simulink model "s_sip_freefall_ss_vs_eom"  (Simulink 6.6)
settings: Solver=ode4  StartTime=0.0  StopTime=3  FixedStep=0.002  RelTol=1e-3  AbsTol=1e-6
values from neighbouring files (symbols this model uses):
  A = handles.A    [d_gui_lqr_tuning.m]
  B = handles.B    [d_gui_lqr_tuning.m]
  Beq = 5.4    [setup_ip01_2_configuration.m]
  C = handles.C    [d_gui_lqr_tuning.m]    (also in d_ip01_2_sip_lqr.m = eye( 4 ))
  D = handles.D    [d_gui_lqr_tuning.m]    (also in d_ip01_2_sip_lqr.m = zeros( 4, 1 ))
  Eff_g = 1    [setup_ip01_2_configuration.m]
  Eff_m = 1    [setup_ip01_2_configuration.m]
  IC_ALPHA0 = IC_ALPHA0 / 180 * pi    (= 0)    [setup_lab_ip01_2_sip.m]
  IMAX_AMP = 1.6    [setup_ip01_2_configuration.m]
  Kg = 3.71    [setup_ip01_2_configuration.m]
  Km = 0.804e-3 * K_RDPS2RPM    [setup_ip01_2_configuration.m]
  Kt = 1.088 * K_OZ2N * K_IN2M    [setup_ip01_2_configuration.m]
  Mc = Mc + Eff_g * Kg^2 * Jm / r_mp^2    [setup_lab_ip01_2_sip.m]
  r_mp = 0.5 / 2 * K_IN2M    [setup_ip01_2_configuration.m]
  Rm = 2.6    [setup_ip01_2_configuration.m]
undefined symbols (not defined in the file or in its folder): Bp, g, Ip, lp, Mp
libraries: simulink_extras x1
settings Model: Creator=MLevis  LastModifiedBy=MLevis  ExtModeTrigDuration=5000  ExtModeArmWhenConnect=off  BufferReuse=off
settings SolverCC: PositivePriorityOrder=on
settings DataIOCC: LimitDataPoints=off
settings OptimizationCC: BooleanDataType=off  OptimizeBlockIOStorage=off  BufferReuse=off  EnforceIntegerDowncast=off  ExpressionFolding=off  FoldNonRolledExpr=off  LocalBlockOutputs=off
settings DebuggingCC: SignalResolutionControl=TryResolveAllWithWarning  SolverPrmCheckMsg=none  MultiTaskDSMMsg=warning  MultiTaskCondExecSysMsg=none  StrictBusMsg=None
settings RTWCC: SystemTargetFile=quarc_windows.tlc  TemplateMakefile=quarc_default_tmf  Description=QUARC Win32 Target  ProcessScript=quarc_windows_make_rtw_hook  IncludeERTFirstTime=on
settings STFCustomTargetCC: TargetFcnLib=ansi_tfl_tmw.mat  TargetPreCompLibLocation=C:\DOCUME~1\ALLUSE~1\APPLIC~1\QUARC\lib\2007a\windows\release  GenFloatMathFcnCalls=ANSI_C  SystemTargetFile=quarc_windows.tlc
settings GRTTargetCC: TargetPreCompLibLocation=C:\DOCUME~1\ALLUSE~1\APPLIC~1\QUARC\lib\2007a\windows\release  MatFileLogging=off  ExtMode=on  ExtModeMexFile=quarc_comm

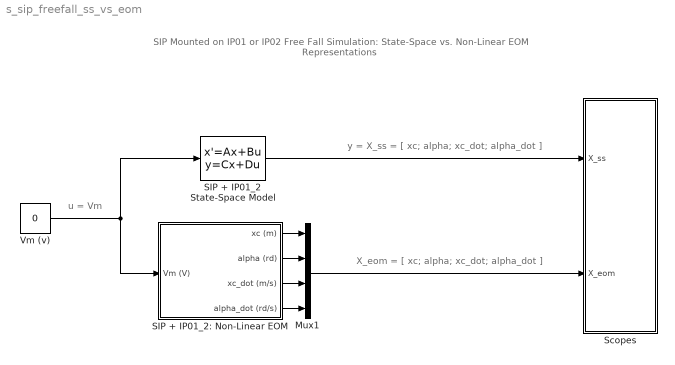
== system s_sip_freefall_ss_vs_eom ==
  note: SIP Mounted on IP01 or IP02
      | Free Fall Simulation:
      | State-Space vs. Non-Linear EOM Representations
  note: u = Vm
  note: y = X_ss = [ xc; alpha; xc_dot; alpha_dot ]
  note: X_eom = [ xc; alpha; xc_dot; alpha_dot ]
  Mux1 : Mux
  SIP + IP01_2 State-Space Model : StateSpace  A=A  B=B  C=C  D=D  X0=[ 0; IC_ALPHA0; 0; 0 ]
  SIP + IP01_2: Non-Linear EOM : Subsystem
  Scopes : Subsystem
  Vm (v) : Constant  Value=0
  wires:
  Vm (v)/1 -> SIP + IP01_2 State-Space Model/1, SIP + IP01_2: Non-Linear EOM/1(Vm (V))
  Mux1/1 -> Scopes/2(X_eom)
  SIP + IP01_2 State-Space Model/1 -> Scopes/1(X_ss)
  SIP + IP01_2: Non-Linear EOM/1(xc (m)) -> Mux1/1
  SIP + IP01_2: Non-Linear EOM/2(alpha (rd)) -> Mux1/2
  SIP + IP01_2: Non-Linear EOM/3(xc_dot (m/s)) -> Mux1/3
  SIP + IP01_2: Non-Linear EOM/4(alpha_dot (rd/s)) -> Mux1/4

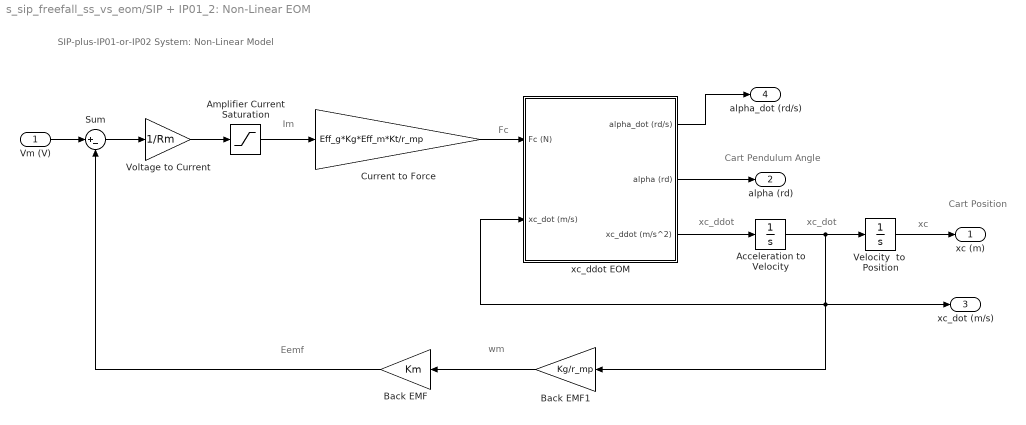
== system s_sip_freefall_ss_vs_eom/SIP + IP01_2: Non-Linear EOM ==
  note: SIP-plus-IP01-or-IP02 System:
      | Non-Linear Model
  note: Fc
  note: Im
  note: Eemf
  note: wm
  note: xc_dot
  note: xc_ddot
  note: xc
  note: Cart Position
  note: Cart Pendulum Angle
  Vm (V) : Inport
  Acceleration to Velocity : Integrator
  Amplifier Current Saturation : Saturate  UpperLimit=IMAX_AMP  LowerLimit=- IMAX_AMP
  Back EMF : Gain  Orientation=left  Gain=Km  SaturateOnIntegerOverflow=on
  Back EMF1 : Gain  Orientation=left  Gain=Kg/r_mp  SaturateOnIntegerOverflow=on
  Current to Force : Gain  Gain=Eff_g*Kg*Eff_m*Kt/r_mp  SaturateOnIntegerOverflow=on
  Sum : Sum  Inputs=|+-  SaturateOnIntegerOverflow=on  InputSameDT=on
  Velocity  to  Position : Integrator
  Voltage to Current : Gain  Gain=1/Rm  SaturateOnIntegerOverflow=on
  xc_ddot EOM : Subsystem
  xc (m) : Outport
  alpha (rd) : Outport  Port=2
  xc_dot (m/s) : Outport  Port=3  InitialOutput=0
  alpha_dot (rd/s) : Outport  Port=4  InitialOutput=0
  wires:
  Sum/1 -> Voltage to Current/1
  Voltage to Current/1 -> Amplifier Current Saturation/1
  Acceleration to Velocity/1 -> xc_dot (m/s)/1, xc_ddot EOM/2(xc_dot (m/s)), Back EMF1/1, Velocity  to  Position/1
  Back EMF1/1 -> Back EMF/1
  Vm (V)/1 -> Sum/1
  Velocity  to  Position/1 -> xc (m)/1
  Back EMF/1 -> Sum/2
  Amplifier Current Saturation/1 -> Current to Force/1
  Current to Force/1 -> xc_ddot EOM/1(Fc (N))
  xc_ddot EOM/3(xc_ddot (m/s^2)) -> Acceleration to Velocity/1
  xc_ddot EOM/1(alpha_dot (rd/s)) -> alpha_dot (rd/s)/1
  xc_ddot EOM/2(alpha (rd)) -> alpha (rd)/1

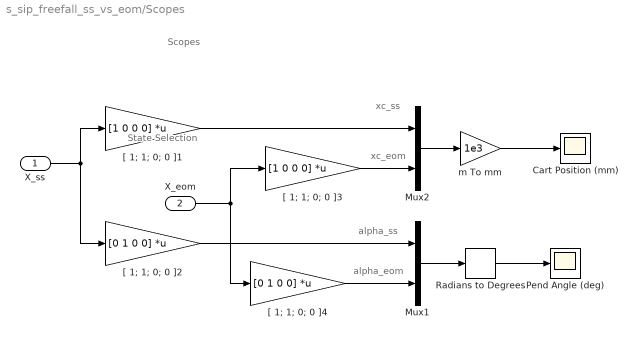
== system s_sip_freefall_ss_vs_eom/Scopes ==
  note: xc_ss
  note: State Selection
  note: alpha_ss
  note: alpha_eom
  note: xc_eom
  note: Scopes
  X_ss : Inport
  X_eom : Inport  Port=2
  Cart Position (mm) : Scope
      settings: TickLabels=on  TimeRange=3  YMin=-50  YMax=50  DataFormat=Array
  Mux1 : Mux  Inputs=2
  Mux2 : Mux  Inputs=2
  Pend Angle (deg) : Scope
      settings: TickLabels=on  TimeRange=3  YMin=-2  YMax=320  DataFormat=Array
  Radians to Degrees : simulink_extras/Transformations/Radians to Degrees  SystemSampleTime=-1
  "[ 1; 1; 0; 0 ]1" : Gain  Gain=[1 0 0 0]  Multiplication=Matrix(K*u)  SaturateOnIntegerOverflow=on
  "[ 1; 1; 0; 0 ]2" : Gain  Gain=[0 1 0 0]  Multiplication=Matrix(K*u)  SaturateOnIntegerOverflow=on
  "[ 1; 1; 0; 0 ]3" : Gain  Gain=[1 0 0 0]  Multiplication=Matrix(K*u)  SaturateOnIntegerOverflow=on
  "[ 1; 1; 0; 0 ]4" : Gain  Gain=[0 1 0 0]  Multiplication=Matrix(K*u)  SaturateOnIntegerOverflow=on
  m To mm : Gain  Gain=1e3  SaturateOnIntegerOverflow=on
  wires:
  Mux2/1 -> m To mm/1
  m To mm/1 -> Cart Position (mm)/1
  X_ss/1 -> "[ 1; 1; 0; 0 ]1"/1, "[ 1; 1; 0; 0 ]2"/1
  Mux1/1 -> Radians to Degrees/1
  Radians to Degrees/1 -> Pend Angle (deg)/1
  X_eom/1 -> "[ 1; 1; 0; 0 ]3"/1, "[ 1; 1; 0; 0 ]4"/1
  "[ 1; 1; 0; 0 ]3"/1 -> Mux2/2
  "[ 1; 1; 0; 0 ]4"/1 -> Mux1/2
  "[ 1; 1; 0; 0 ]2"/1 -> Mux1/1
  "[ 1; 1; 0; 0 ]1"/1 -> Mux2/1

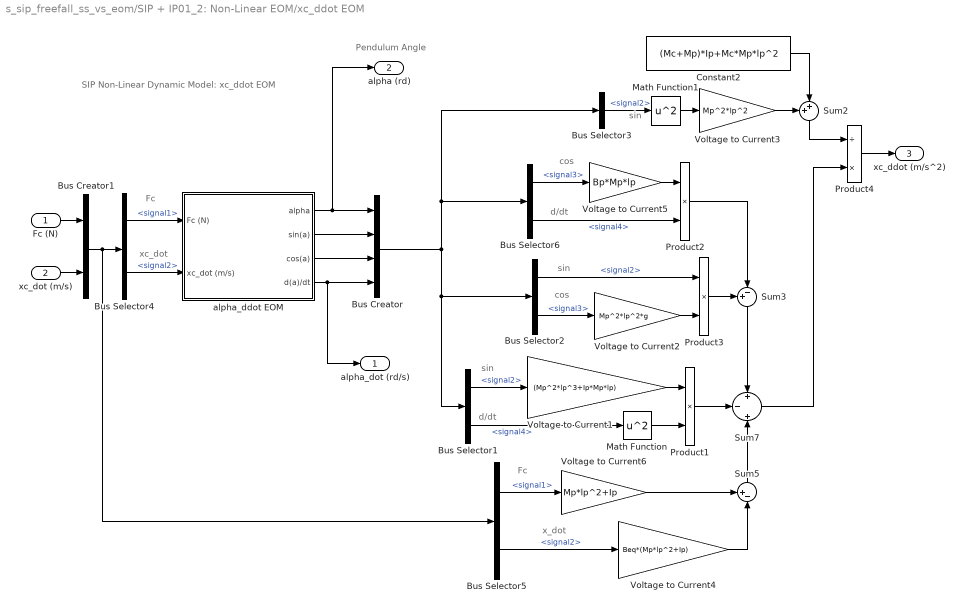
== system s_sip_freefall_ss_vs_eom/SIP + IP01_2: Non-Linear EOM/xc_ddot EOM ==
  note: xc_dot
  note: Fc
  note: x_dot
  note: Fc
  note: d/dt
  note: cos
  note: Pendulum Angle
  note: sin
  note: cos
  note: sin
  note: sin
  note: d/dt
  note: SIP Non-Linear Dynamic Model:
      | xc_ddot EOM
  Fc (N) : Inport
  xc_dot (m/s) : Inport  Port=2
  Bus Creator : BusCreator
  Bus Creator1 : BusCreator  Inputs=2
  Bus Selector1 : BusSelector  OutputSignals=signal2,signal4
  Bus Selector2 : BusSelector  OutputSignals=signal2,signal3
  Bus Selector3 : BusSelector  OutputSignals=signal2
  Bus Selector4 : BusSelector  OutputSignals=signal1,signal2
  Bus Selector5 : BusSelector  OutputSignals=signal1,signal2
  Bus Selector6 : BusSelector  OutputSignals=signal3,signal4
  Constant2 : Constant  Value=(Mc+Mp)*Ip+Mc*Mp*lp^2
  Math Function : Math  Operator=square  SaturateOnIntegerOverflow=on
  Math Function1 : Math  Operator=square  SaturateOnIntegerOverflow=on
  Product1 : Product  SaturateOnIntegerOverflow=on  RndMeth=Zero  InputSameDT=on
  Product2 : Product  SaturateOnIntegerOverflow=on  RndMeth=Zero  InputSameDT=on
  Product3 : Product  SaturateOnIntegerOverflow=on  RndMeth=Zero  InputSameDT=on
  Product4 : Product  Inputs=/*  SaturateOnIntegerOverflow=on  RndMeth=Zero  InputSameDT=on
  Sum2 : Sum  Orientation=down  Inputs=++|  SaturateOnIntegerOverflow=on  InputSameDT=on
  Sum3 : Sum  Orientation=down  Inputs=+-|  SaturateOnIntegerOverflow=on  InputSameDT=on
  Sum5 : Sum  Orientation=up  Inputs=+-|  SaturateOnIntegerOverflow=on  InputSameDT=on
  Sum7 : Sum  Inputs=+|-|+  SaturateOnIntegerOverflow=on  InputSameDT=on
  Voltage to Current1 : Gain  Gain=(Mp^2*lp^3+Ip*Mp*lp)  SaturateOnIntegerOverflow=on
  Voltage to Current2 : Gain  Gain=Mp^2*lp^2*g  SaturateOnIntegerOverflow=on
  Voltage to Current3 : Gain  Gain=Mp^2*lp^2  SaturateOnIntegerOverflow=on
  Voltage to Current4 : Gain  Gain=Beq*(Mp*lp^2+Ip)  SaturateOnIntegerOverflow=on
  Voltage to Current5 : Gain  Gain=Bp*Mp*lp  SaturateOnIntegerOverflow=on
  Voltage to Current6 : Gain  Gain=Mp*lp^2+Ip  SaturateOnIntegerOverflow=on
  alpha_ddot EOM : Subsystem
  alpha_dot (rd/s) : Outport
  alpha (rd) : Outport  Port=2
  xc_ddot (m/s^2) : Outport  Port=3
  wires:
  Voltage to Current4/1 -> Sum5/2
  Voltage to Current6/1 -> Sum5/1
  Sum5/1 -> Sum7/3
  Sum3/1 -> Sum7/1
  Product3/1 -> Sum3/1
  Product2/1 -> Sum3/2
  Sum7/1 -> Product4/2
  Bus Selector5/2 -> Voltage to Current4/1  "<signal2>"
  Bus Selector5/1 -> Voltage to Current6/1  "<signal1>"
  Voltage to Current5/1 -> Product2/1
  Bus Selector2/2 -> Voltage to Current2/1  "<signal3>"
  Bus Selector2/1 -> Product3/1  "<signal2>"
  Bus Selector6/2 -> Product2/2  "<signal4>"
  Bus Selector6/1 -> Voltage to Current5/1  "<signal3>"
  Bus Selector1/1 -> Voltage to Current1/1  "<signal2>"
  Bus Selector1/2 -> Math Function/1  "<signal4>"
  Bus Selector4/2 -> alpha_ddot EOM/2(xc_dot (m/s))  "<signal2>"
  Bus Selector4/1 -> alpha_ddot EOM/1(Fc (N))  "<signal1>"
  Bus Creator1/1 -> Bus Selector5/1, Bus Selector4/1
  xc_dot (m/s)/1 -> Bus Creator1/2
  Fc (N)/1 -> Bus Creator1/1
  alpha_ddot EOM/4(d(a)/dt) -> Bus Creator/4, alpha_dot (rd/s)/1
  alpha_ddot EOM/3(cos(a)) -> Bus Creator/3
  alpha_ddot EOM/2(sin(a)) -> Bus Creator/2
  alpha_ddot EOM/1(alpha) -> alpha (rd)/1, Bus Creator/1
  Product4/1 -> xc_ddot (m/s^2)/1
  Product1/1 -> Sum7/2
  Constant2/1 -> Sum2/2
  Voltage to Current3/1 -> Sum2/1
  Math Function1/1 -> Voltage to Current3/1
  Bus Selector3/1 -> Math Function1/1  "<signal2>"
  Voltage to Current2/1 -> Product3/2
  Math Function/1 -> Product1/2
  Voltage to Current1/1 -> Product1/1
  Bus Creator/1 -> Bus Selector6/1, Bus Selector3/1, Bus Selector1/1, Bus Selector2/1
  Sum2/1 -> Product4/1

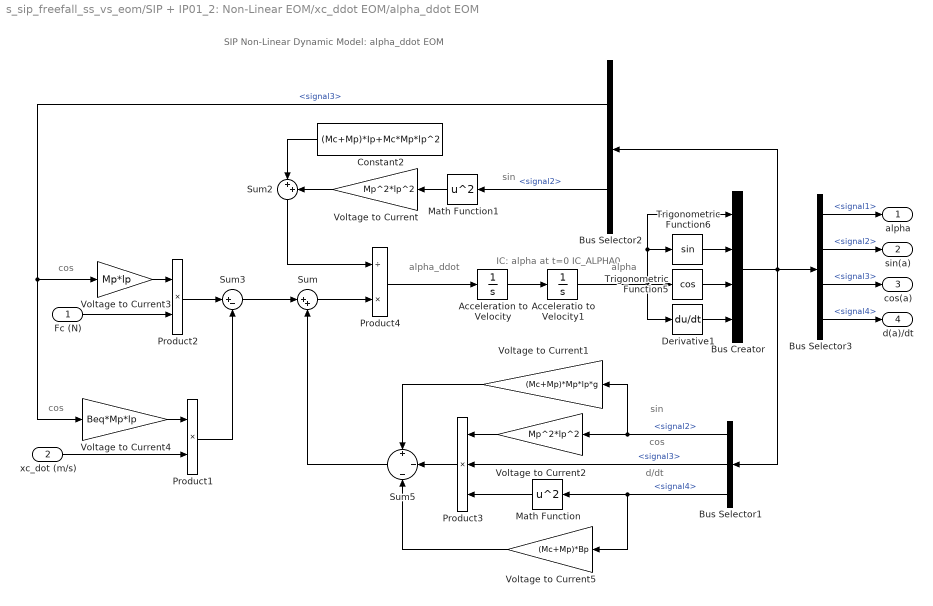
== system s_sip_freefall_ss_vs_eom/SIP + IP01_2: Non-Linear EOM/xc_ddot EOM/alpha_ddot EOM ==
  note: cos
  note: alpha_ddot
  note: IC: alpha at t=0
      | IC_ALPHA0
  note: SIP Non-Linear Dynamic Model:
      | alpha_ddot EOM
  note: alpha
  note: sin
  note: cos
  note: sin
  note: cos
  note: d/dt
  Fc (N) : Inport
  xc_dot (m/s) : Inport  Port=2
  Acceleratio to Velocity1 : Integrator  InitialCondition=IC_ALPHA0
  Acceleration to Velocity : Integrator
  Bus Creator : BusCreator
  Bus Selector1 : BusSelector  Orientation=left  OutputSignals=signal2,signal3,signal4
  Bus Selector2 : BusSelector  Orientation=left  OutputSignals=signal3,signal2
  Bus Selector3 : BusSelector  OutputSignals=signal1,signal2,signal3,signal4
  Constant2 : Constant  Orientation=left  Value=(Mc+Mp)*Ip+Mc*Mp*lp^2
  Derivative1 : Derivative
  Math Function : Math  Orientation=left  Operator=square  SaturateOnIntegerOverflow=on
  Math Function1 : Math  Orientation=left  Operator=square  SaturateOnIntegerOverflow=on
  Product1 : Product  SaturateOnIntegerOverflow=on  RndMeth=Zero  InputSameDT=on
  Product2 : Product  SaturateOnIntegerOverflow=on  RndMeth=Zero  InputSameDT=on
  Product3 : Product  Orientation=left  Inputs=3  SaturateOnIntegerOverflow=on  RndMeth=Zero  InputSameDT=on
  Product4 : Product  Inputs=/*  SaturateOnIntegerOverflow=on  RndMeth=Zero  InputSameDT=on
  Sum : Sum  Inputs=|++  SaturateOnIntegerOverflow=on  InputSameDT=on
  Sum2 : Sum  Orientation=down  Inputs=|++  SaturateOnIntegerOverflow=on  InputSameDT=on
  Sum3 : Sum  Inputs=|+-  SaturateOnIntegerOverflow=on  InputSameDT=on
  Sum5 : Sum  Orientation=left  Inputs=+|-|-  SaturateOnIntegerOverflow=on  InputSameDT=on
  Trigonometric Function5 : Trigonometry  Operator=cos
  Trigonometric Function6 : Trigonometry
  Voltage to Current : Gain  Orientation=left  Gain=Mp^2*lp^2  SaturateOnIntegerOverflow=on
  Voltage to Current1 : Gain  Orientation=left  Gain=(Mc+Mp)*Mp*lp*g  SaturateOnIntegerOverflow=on
  Voltage to Current2 : Gain  Orientation=left  Gain=Mp^2*lp^2  SaturateOnIntegerOverflow=on
  Voltage to Current3 : Gain  Gain=Mp*lp  SaturateOnIntegerOverflow=on
  Voltage to Current4 : Gain  Gain=Beq*Mp*lp  SaturateOnIntegerOverflow=on
  Voltage to Current5 : Gain  Orientation=left  Gain=(Mc+Mp)*Bp  SaturateOnIntegerOverflow=on
  alpha : Outport  InitialOutput=0
  sin(a) : Outport  Port=2  InitialOutput=0
  cos(a) : Outport  Port=3  InitialOutput=0
  d(a)/dt : Outport  Port=4  InitialOutput=0
  wires:
  Sum5/1 -> Sum/2
  Voltage to Current5/1 -> Sum5/3
  Voltage to Current1/1 -> Sum5/1
  Product3/1 -> Sum5/2
  Sum3/1 -> Sum/1
  Product1/1 -> Sum3/2
  Product2/1 -> Sum3/1
  Voltage to Current4/1 -> Product1/1
  xc_dot (m/s)/1 -> Product1/2
  Fc (N)/1 -> Product2/2
  Voltage to Current3/1 -> Product2/1
  Acceleratio to Velocity1/1 -> Bus Creator/1, Trigonometric Function6/1, Derivative1/1, Trigonometric Function5/1
  Bus Selector3/4 -> d(a)/dt/1  "<signal4>"
  Bus Selector3/3 -> cos(a)/1  "<signal3>"
  Bus Selector3/2 -> sin(a)/1  "<signal2>"
  Bus Selector3/1 -> alpha/1  "<signal1>"
  Bus Selector1/3 -> Voltage to Current5/1, Math Function/1  "<signal4>"
  Bus Selector1/2 -> Product3/2  "<signal3>"
  Voltage to Current2/1 -> Product3/1
  Bus Selector2/1 -> Voltage to Current4/1, Voltage to Current3/1  "<signal3>"
  Bus Creator/1 -> Bus Selector3/1, Bus Selector1/1, Bus Selector2/1
  Derivative1/1 -> Bus Creator/4
  Trigonometric Function5/1 -> Bus Creator/3
  Trigonometric Function6/1 -> Bus Creator/2
  Constant2/1 -> Sum2/1
  Math Function1/1 -> Voltage to Current/1
  Bus Selector2/2 -> Math Function1/1  "<signal2>"
  Voltage to Current/1 -> Sum2/2
  Sum/1 -> Product4/2
  Sum2/1 -> Product4/1
  Math Function/1 -> Product3/3
  Product4/1 -> Acceleration to Velocity/1
  Bus Selector1/1 -> Voltage to Current2/1, Voltage to Current1/1  "<signal2>"
  Acceleration to Velocity/1 -> Acceleratio to Velocity1/1
